simulink model "ALL_JP360_DBW_V6_5_1103"  (R2022a)
settings: Solver=FixedStepAuto  StartTime=0.0  StopTime=inf  FixedStep=0.01  RelTol=1e-3  EnableMultiTasking=on
model workspace (MAT data in the model file):
  g = 9.8
undefined symbols (not defined in the file or in its folder): canChannel, delta_v_p, IPM_Line_C0, IPM_Line_C1, IPM_Line_C2, IPM_Line_C3, M, M_p, MRR_ObjDistX, MRR_ObjDistY, MRR_ObjFusionCamID, MRR_ObjFusionSig, MRR_ObjID, MRR_ObjRelVelX, MRR_ObjRelVelY, MRR_ObjType, MRR_ObjUpdFlg, none, obj_vaild, untracktime, V, videoinput
libraries: canfdmsglib x230, canfdlib x76, slpidlib x24, simulink x18, dspstat3 x14, ctrlSharedLib x1, simulink_extras x1, imaqlib x1, realtime_pacer_lib x1, dspvision x1, visionsinks x1
(part 48 of 55)

== system ALL_JP360_DBW_V6_5_1103/MsgFromCAN/VR_ADCU_MsgFromCAN/VR_ADCU_MRR_Obj_25_26_0x69C ==
  VR_ADCU_MRR_Obj_25_26_0x69CFromInData : Inport  OutDataTypeStr=Bus:CAN_FD_MESSAGE_BUS
  Bus Creator : BusCreator  Inputs=30  OutDataTypeStr=Bus:VR_ADCU_MRR_Obj_25_26_0x69C  NonVirtualBus=on
  CAN FD Unpack : canfdmsglib/CAN FD Unpack  CANdbFile=HiFire_T360_P789_1R1V_Pri_Matrix_CAN_V2.3_20220810.dbc  MsgList=(none)  MsgName=MRR_Obj_25_26_0x69C  ProtocolMode=CAN FD  MsgIDType=Standard (11-bit identifier)  MsgIdentifier=1692  MsgLength=32  SignalInfo={'MRR_ObjDistX_25','26','12','BE','unsigned','Standard','0','0.0625','0','0','254.9375';'MRR_ObjDistX_26','130','12','BE','unsigned','Standard','0','0.0625','0','0','254.9375';'MRR_ObjDistY_25','44','14','BE','unsigned','Standard','0','0.0078125','-64','-64','63.9922';'MRR_ObjDistY_26','148','14','BE','unsigned','Standard','0','0.0078125','-64','-64','63.9922';'MRR_ObjExistProb_25','11','5','BE','unsigned','Standard','0','0.03125','0','0','0.96875';'MRR_ObjExistProb_26','115','5','BE','unsigned','Standard','0','0.03125','0','0','0.96875';'MRR_ObjFusionCamID_25','208','8','BE','unsigned','Standard','0','1','0','0','255';'MRR_ObjFusionCamID_26','216','8','BE','unsigned','Standard','0','1','0','0','255';'MRR_ObjFusionSig_25','98','2','BE','unsigned','Standard','0','1','0','0','3';'MRR_ObjFusionSig_26','202','2','BE','unsigned','Standard','0','1','0','0','3';'MRR_ObjID_25','0','8','BE','unsigned','Standard','0','1','0','0','255';'MRR_ObjID_26','104','8','BE','unsigned','Standard','0','1','0','0','255';'MRR_ObjMovingSts_25','103','3','BE','unsigned','Standard','0','1','0','0','7';'MRR_ObjMovingSts_26','207','3','BE','unsigned','Standard','0','1','0','0','7';'MRR_ObjObstacleProb_25','22','5','BE','unsigned','Standard','0','0.03125','0','0','0.96875';'MRR_ObjObstacleProb_26','126','5','BE','unsigned','Standard','0','0.03125','0','0','0.96875';'MRR_ObjRelAccelX_25','72','10','BE','unsigned','Standard','0','0.03125','-16','-16','15.9688';'MRR_ObjRelAccelX_26','176','10','BE','unsigned','Standard','0','0.03125','-16','-16','15.9688';'MRR_ObjRelAccelY_25','94','10','BE','unsigned','Standard','0','0.03125','-16','-16','15.9688';'MRR_ObjRelAccelY_26','198','10','BE','unsigned','Standard','0','0.03125','-16','-16','15.9688';'MRR_ObjRelVelX_25','63','13','BE','unsigned','Standard','0','0.03125','-128','-128','127.9688';'MRR_ObjRelVelX_26','167','13','BE','unsigned','Standard','0','0.03125','-128','-128','127.9688';'MRR_ObjRelVelY_25','66','13','BE','unsigned','Standard','0','0.03125','-128','-128','127.9688';'MRR_ObjRelVelY_26','170','13','BE','unsigned','Standard','0','0.03125','-128','-128','127.9688';'MRR_ObjType_25','90','4','BE','unsigned','Standard','0','1','0','0','15';'MRR_ObjType_26','194','4','BE','unsigned','Standard','0','1','0','0','15';'MRR_ObjUpdFlg_25','100','3','BE','unsigned','Standard','0','1','0','0','7';'MRR_ObjUpdFlg_26','204','3','BE','unsigned','Standard','0','1','0','0','7';'MRR_Obj_25_26_Checksum','248','16','BE','unsigned','Standard','0','1','0','0','65535';'MRR_Obj_25_26_MsgCounter','232','4','BE','unsigned','Standard','0','1','0','0','15'}  IDPort=off  TimestampPort=off  ErrorPort=off  RemotePort=off  LengthPort=off  StatusPort=off  BRSPort=off  ESIPort=off  DLCPort=off  ApplyMinMax=off
      settings: SourceProductBaseCode=ME,XP,VN  DataFormat=CANdb specified signals
  Data Type Conversion{1..6,15..24} (16 alike) : DataTypeConversion  OutDataTypeStr=single  SaturateOnIntegerOverflow=off  RndMeth=Floor
  Data Type Conversion{9..10,13..14,25..28,30} (9 alike) : DataTypeConversion  OutDataTypeStr=int8  SaturateOnIntegerOverflow=off  RndMeth=Floor
  Data Type Conversion{7..8,11..12} (4 alike) : DataTypeConversion  OutDataTypeStr=uint8  SaturateOnIntegerOverflow=off  RndMeth=Floor
  Data Type Conversion29 : DataTypeConversion  OutDataTypeStr=uint16  SaturateOnIntegerOverflow=off  RndMeth=Floor
  VR_ADCU_MRR_Obj_25_26_0x69CFromOutData : Outport  OutDataTypeStr=Bus:VR_ADCU_MRR_Obj_25_26_0x69C
  wires:
  CAN FD Unpack/1 -> Data Type Conversion1/1
  CAN FD Unpack/2 -> Data Type Conversion2/1
  CAN FD Unpack/3 -> Data Type Conversion3/1
  CAN FD Unpack/4 -> Data Type Conversion4/1
  CAN FD Unpack/5 -> Data Type Conversion5/1
  CAN FD Unpack/6 -> Data Type Conversion6/1
  CAN FD Unpack/7 -> Data Type Conversion7/1
  CAN FD Unpack/8 -> Data Type Conversion8/1
  CAN FD Unpack/9 -> Data Type Conversion9/1
  CAN FD Unpack/10 -> Data Type Conversion10/1
  CAN FD Unpack/11 -> Data Type Conversion11/1
  CAN FD Unpack/12 -> Data Type Conversion12/1
  CAN FD Unpack/13 -> Data Type Conversion13/1
  CAN FD Unpack/14 -> Data Type Conversion14/1
  CAN FD Unpack/15 -> Data Type Conversion15/1
  CAN FD Unpack/16 -> Data Type Conversion16/1
  CAN FD Unpack/17 -> Data Type Conversion17/1
  CAN FD Unpack/18 -> Data Type Conversion18/1
  CAN FD Unpack/19 -> Data Type Conversion19/1
  CAN FD Unpack/20 -> Data Type Conversion20/1
  CAN FD Unpack/21 -> Data Type Conversion21/1
  CAN FD Unpack/22 -> Data Type Conversion22/1
  CAN FD Unpack/23 -> Data Type Conversion23/1
  CAN FD Unpack/24 -> Data Type Conversion24/1
  CAN FD Unpack/25 -> Data Type Conversion25/1
  CAN FD Unpack/26 -> Data Type Conversion26/1
  CAN FD Unpack/27 -> Data Type Conversion27/1
  CAN FD Unpack/28 -> Data Type Conversion28/1
  CAN FD Unpack/29 -> Data Type Conversion29/1
  CAN FD Unpack/30 -> Data Type Conversion30/1
  Data Type Conversion1/1 -> Bus Creator/1  "MRR_ObjDistX_25"
  Data Type Conversion2/1 -> Bus Creator/2  "MRR_ObjDistX_26"
  Data Type Conversion3/1 -> Bus Creator/3  "MRR_ObjDistY_25"
  Data Type Conversion4/1 -> Bus Creator/4  "MRR_ObjDistY_26"
  Data Type Conversion5/1 -> Bus Creator/5  "MRR_ObjExistProb_25"
  Data Type Conversion6/1 -> Bus Creator/6  "MRR_ObjExistProb_26"
  Data Type Conversion7/1 -> Bus Creator/7  "MRR_ObjFusionCamID_25"
  Data Type Conversion8/1 -> Bus Creator/8  "MRR_ObjFusionCamID_26"
  Data Type Conversion9/1 -> Bus Creator/9  "MRR_ObjFusionSig_25"
  Data Type Conversion10/1 -> Bus Creator/10  "MRR_ObjFusionSig_26"
  Data Type Conversion11/1 -> Bus Creator/11  "MRR_ObjID_25"
  Data Type Conversion12/1 -> Bus Creator/12  "MRR_ObjID_26"
  Data Type Conversion13/1 -> Bus Creator/13  "MRR_ObjMovingSts_25"
  Data Type Conversion14/1 -> Bus Creator/14  "MRR_ObjMovingSts_26"
  Data Type Conversion15/1 -> Bus Creator/15  "MRR_ObjObstacleProb_25"
  Data Type Conversion16/1 -> Bus Creator/16  "MRR_ObjObstacleProb_26"
  Data Type Conversion17/1 -> Bus Creator/17  "MRR_ObjRelAccelX_25"
  Data Type Conversion18/1 -> Bus Creator/18  "MRR_ObjRelAccelX_26"
  Data Type Conversion19/1 -> Bus Creator/19  "MRR_ObjRelAccelY_25"
  Data Type Conversion20/1 -> Bus Creator/20  "MRR_ObjRelAccelY_26"
  Data Type Conversion21/1 -> Bus Creator/21  "MRR_ObjRelVelX_25"
  Data Type Conversion22/1 -> Bus Creator/22  "MRR_ObjRelVelX_26"
  Data Type Conversion23/1 -> Bus Creator/23  "MRR_ObjRelVelY_25"
  Data Type Conversion24/1 -> Bus Creator/24  "MRR_ObjRelVelY_26"
  Data Type Conversion25/1 -> Bus Creator/25  "MRR_ObjType_25"
  Data Type Conversion26/1 -> Bus Creator/26  "MRR_ObjType_26"
  Data Type Conversion27/1 -> Bus Creator/27  "MRR_ObjUpdFlg_25"
  Data Type Conversion28/1 -> Bus Creator/28  "MRR_ObjUpdFlg_26"
  Data Type Conversion29/1 -> Bus Creator/29  "MRR_Obj_25_26_Checksum"
  Data Type Conversion30/1 -> Bus Creator/30  "MRR_Obj_25_26_MsgCounter"
  Bus Creator/1 -> VR_ADCU_MRR_Obj_25_26_0x69CFromOutData/1  "VR_ADCU_MRR_Obj_25_26_0x69CFromOutData"
  VR_ADCU_MRR_Obj_25_26_0x69CFromInData/1 -> CAN FD Unpack/1  "VR_ADCU_MRR_Obj_25_26_0x69CFromInData"

== system ALL_JP360_DBW_V6_5_1103/MsgFromCAN/VR_ADCU_MsgFromCAN/VR_ADCU_MRR_Obj_27_28_0x69D ==
  VR_ADCU_MRR_Obj_27_28_0x69DFromInData : Inport  OutDataTypeStr=Bus:CAN_FD_MESSAGE_BUS
  Bus Creator : BusCreator  Inputs=30  OutDataTypeStr=Bus:VR_ADCU_MRR_Obj_27_28_0x69D  NonVirtualBus=on
  CAN FD Unpack : canfdmsglib/CAN FD Unpack  CANdbFile=HiFire_T360_P789_1R1V_Pri_Matrix_CAN_V2.3_20220810.dbc  MsgList=(none)  MsgName=MRR_Obj_27_28_0x69D  ProtocolMode=CAN FD  MsgIDType=Standard (11-bit identifier)  MsgIdentifier=1693  MsgLength=32  SignalInfo={'MRR_ObjDistX_27','26','12','BE','unsigned','Standard','0','0.0625','0','0','254.9375';'MRR_ObjDistX_28','130','12','BE','unsigned','Standard','0','0.0625','0','0','254.9375';'MRR_ObjDistY_27','44','14','BE','unsigned','Standard','0','0.0078125','-64','-64','63.9922';'MRR_ObjDistY_28','148','14','BE','unsigned','Standard','0','0.0078125','-64','-64','63.9922';'MRR_ObjExistProb_27','11','5','BE','unsigned','Standard','0','0.03125','0','0','0.96875';'MRR_ObjExistProb_28','115','5','BE','unsigned','Standard','0','0.03125','0','0','0.96875';'MRR_ObjFusionCamID_27','208','8','BE','unsigned','Standard','0','1','0','0','255';'MRR_ObjFusionCamID_28','216','8','BE','unsigned','Standard','0','1','0','0','255';'MRR_ObjFusionSig_27','98','2','BE','unsigned','Standard','0','1','0','0','3';'MRR_ObjFusionSig_28','202','2','BE','unsigned','Standard','0','1','0','0','3';'MRR_ObjID_27','0','8','BE','unsigned','Standard','0','1','0','0','255';'MRR_ObjID_28','104','8','BE','unsigned','Standard','0','1','0','0','255';'MRR_ObjMovingSts_27','103','3','BE','unsigned','Standard','0','1','0','0','7';'MRR_ObjMovingSts_28','207','3','BE','unsigned','Standard','0','1','0','0','7';'MRR_ObjObstacleProb_27','22','5','BE','unsigned','Standard','0','0.03125','0','0','0.96875';'MRR_ObjObstacleProb_28','126','5','BE','unsigned','Standard','0','0.03125','0','0','0.96875';'MRR_ObjRelAccelX_27','72','10','BE','unsigned','Standard','0','0.03125','-16','-16','15.9688';'MRR_ObjRelAccelX_28','176','10','BE','unsigned','Standard','0','0.03125','-16','-16','15.9688';'MRR_ObjRelAccelY_27','94','10','BE','unsigned','Standard','0','0.03125','-16','-16','15.9688';'MRR_ObjRelAccelY_28','198','10','BE','unsigned','Standard','0','0.03125','-16','-16','15.9688';'MRR_ObjRelVelX_27','63','13','BE','unsigned','Standard','0','0.03125','-128','-128','127.9688';'MRR_ObjRelVelX_28','167','13','BE','unsigned','Standard','0','0.03125','-128','-128','127.9688';'MRR_ObjRelVelY_27','66','13','BE','unsigned','Standard','0','0.03125','-128','-128','127.9688';'MRR_ObjRelVelY_28','170','13','BE','unsigned','Standard','0','0.03125','-128','-128','127.9688';'MRR_ObjType_27','90','4','BE','unsigned','Standard','0','1','0','0','15';'MRR_ObjType_28','194','4','BE','unsigned','Standard','0','1','0','0','15';'MRR_ObjUpdFlg_27','100','3','BE','unsigned','Standard','0','1','0','0','7';'MRR_ObjUpdFlg_28','204','3','BE','unsigned','Standard','0','1','0','0','7';'MRR_Obj_27_28_Checksum','248','16','BE','unsigned','Standard','0','1','0','0','65535';'MRR_Obj_27_28_MsgCounter','232','4','BE','unsigned','Standard','0','1','0','0','15'}  IDPort=off  TimestampPort=off  ErrorPort=off  RemotePort=off  LengthPort=off  StatusPort=off  BRSPort=off  ESIPort=off  DLCPort=off  ApplyMinMax=off
      settings: SourceProductBaseCode=ME,XP,VN  DataFormat=CANdb specified signals
  Data Type Conversion{1..6,15..24} (16 alike) : DataTypeConversion  OutDataTypeStr=single  SaturateOnIntegerOverflow=off  RndMeth=Floor
  Data Type Conversion{9..10,13..14,25..28,30} (9 alike) : DataTypeConversion  OutDataTypeStr=int8  SaturateOnIntegerOverflow=off  RndMeth=Floor
  Data Type Conversion{7..8,11..12} (4 alike) : DataTypeConversion  OutDataTypeStr=uint8  SaturateOnIntegerOverflow=off  RndMeth=Floor
  Data Type Conversion29 : DataTypeConversion  OutDataTypeStr=uint16  SaturateOnIntegerOverflow=off  RndMeth=Floor
  VR_ADCU_MRR_Obj_27_28_0x69DFromOutData : Outport  OutDataTypeStr=Bus:VR_ADCU_MRR_Obj_27_28_0x69D
  wires:
  CAN FD Unpack/1 -> Data Type Conversion1/1
  CAN FD Unpack/2 -> Data Type Conversion2/1
  CAN FD Unpack/3 -> Data Type Conversion3/1
  CAN FD Unpack/4 -> Data Type Conversion4/1
  CAN FD Unpack/5 -> Data Type Conversion5/1
  CAN FD Unpack/6 -> Data Type Conversion6/1
  CAN FD Unpack/7 -> Data Type Conversion7/1
  CAN FD Unpack/8 -> Data Type Conversion8/1
  CAN FD Unpack/9 -> Data Type Conversion9/1
  CAN FD Unpack/10 -> Data Type Conversion10/1
  CAN FD Unpack/11 -> Data Type Conversion11/1
  CAN FD Unpack/12 -> Data Type Conversion12/1
  CAN FD Unpack/13 -> Data Type Conversion13/1
  CAN FD Unpack/14 -> Data Type Conversion14/1
  CAN FD Unpack/15 -> Data Type Conversion15/1
  CAN FD Unpack/16 -> Data Type Conversion16/1
  CAN FD Unpack/17 -> Data Type Conversion17/1
  CAN FD Unpack/18 -> Data Type Conversion18/1
  CAN FD Unpack/19 -> Data Type Conversion19/1
  CAN FD Unpack/20 -> Data Type Conversion20/1
  CAN FD Unpack/21 -> Data Type Conversion21/1
  CAN FD Unpack/22 -> Data Type Conversion22/1
  CAN FD Unpack/23 -> Data Type Conversion23/1
  CAN FD Unpack/24 -> Data Type Conversion24/1
  CAN FD Unpack/25 -> Data Type Conversion25/1
  CAN FD Unpack/26 -> Data Type Conversion26/1
  CAN FD Unpack/27 -> Data Type Conversion27/1
  CAN FD Unpack/28 -> Data Type Conversion28/1
  CAN FD Unpack/29 -> Data Type Conversion29/1
  CAN FD Unpack/30 -> Data Type Conversion30/1
  Data Type Conversion1/1 -> Bus Creator/1  "MRR_ObjDistX_27"
  Data Type Conversion2/1 -> Bus Creator/2  "MRR_ObjDistX_28"
  Data Type Conversion3/1 -> Bus Creator/3  "MRR_ObjDistY_27"
  Data Type Conversion4/1 -> Bus Creator/4  "MRR_ObjDistY_28"
  Data Type Conversion5/1 -> Bus Creator/5  "MRR_ObjExistProb_27"
  Data Type Conversion6/1 -> Bus Creator/6  "MRR_ObjExistProb_28"
  Data Type Conversion7/1 -> Bus Creator/7  "MRR_ObjFusionCamID_27"
  Data Type Conversion8/1 -> Bus Creator/8  "MRR_ObjFusionCamID_28"
  Data Type Conversion9/1 -> Bus Creator/9  "MRR_ObjFusionSig_27"
  Data Type Conversion10/1 -> Bus Creator/10  "MRR_ObjFusionSig_28"
  Data Type Conversion11/1 -> Bus Creator/11  "MRR_ObjID_27"
  Data Type Conversion12/1 -> Bus Creator/12  "MRR_ObjID_28"
  Data Type Conversion13/1 -> Bus Creator/13  "MRR_ObjMovingSts_27"
  Data Type Conversion14/1 -> Bus Creator/14  "MRR_ObjMovingSts_28"
  Data Type Conversion15/1 -> Bus Creator/15  "MRR_ObjObstacleProb_27"
  Data Type Conversion16/1 -> Bus Creator/16  "MRR_ObjObstacleProb_28"
  Data Type Conversion17/1 -> Bus Creator/17  "MRR_ObjRelAccelX_27"
  Data Type Conversion18/1 -> Bus Creator/18  "MRR_ObjRelAccelX_28"
  Data Type Conversion19/1 -> Bus Creator/19  "MRR_ObjRelAccelY_27"
  Data Type Conversion20/1 -> Bus Creator/20  "MRR_ObjRelAccelY_28"
  Data Type Conversion21/1 -> Bus Creator/21  "MRR_ObjRelVelX_27"
  Data Type Conversion22/1 -> Bus Creator/22  "MRR_ObjRelVelX_28"
  Data Type Conversion23/1 -> Bus Creator/23  "MRR_ObjRelVelY_27"
  Data Type Conversion24/1 -> Bus Creator/24  "MRR_ObjRelVelY_28"
  Data Type Conversion25/1 -> Bus Creator/25  "MRR_ObjType_27"
  Data Type Conversion26/1 -> Bus Creator/26  "MRR_ObjType_28"
  Data Type Conversion27/1 -> Bus Creator/27  "MRR_ObjUpdFlg_27"
  Data Type Conversion28/1 -> Bus Creator/28  "MRR_ObjUpdFlg_28"
  Data Type Conversion29/1 -> Bus Creator/29  "MRR_Obj_27_28_Checksum"
  Data Type Conversion30/1 -> Bus Creator/30  "MRR_Obj_27_28_MsgCounter"
  Bus Creator/1 -> VR_ADCU_MRR_Obj_27_28_0x69DFromOutData/1  "VR_ADCU_MRR_Obj_27_28_0x69DFromOutData"
  VR_ADCU_MRR_Obj_27_28_0x69DFromInData/1 -> CAN FD Unpack/1  "VR_ADCU_MRR_Obj_27_28_0x69DFromInData"

== system ALL_JP360_DBW_V6_5_1103/MsgFromCAN/VR_ADCU_MsgFromCAN/VR_ADCU_MRR_Obj_29_30_0x69E ==
  VR_ADCU_MRR_Obj_29_30_0x69EFromInData : Inport  OutDataTypeStr=Bus:CAN_FD_MESSAGE_BUS
  Bus Creator : BusCreator  Inputs=30  OutDataTypeStr=Bus:VR_ADCU_MRR_Obj_29_30_0x69E  NonVirtualBus=on
  CAN FD Unpack : canfdmsglib/CAN FD Unpack  CANdbFile=HiFire_T360_P789_1R1V_Pri_Matrix_CAN_V2.3_20220810.dbc  MsgList=(none)  MsgName=MRR_Obj_29_30_0x69E  ProtocolMode=CAN FD  MsgIDType=Standard (11-bit identifier)  MsgIdentifier=1694  MsgLength=32  SignalInfo={'MRR_ObjDistX_29','26','12','BE','unsigned','Standard','0','0.0625','0','0','254.9375';'MRR_ObjDistX_30','130','12','BE','unsigned','Standard','0','0.0625','0','0','254.9375';'MRR_ObjDistY_29','44','14','BE','unsigned','Standard','0','0.0078125','-64','-64','63.9922';'MRR_ObjDistY_30','148','14','BE','unsigned','Standard','0','0.0078125','-64','-64','63.9922';'MRR_ObjExistProb_29','11','5','BE','unsigned','Standard','0','0.03125','0','0','0.96875';'MRR_ObjExistProb_30','115','5','BE','unsigned','Standard','0','0.03125','0','0','0.96875';'MRR_ObjFusionCamID_29','208','8','BE','unsigned','Standard','0','1','0','0','255';'MRR_ObjFusionCamID_30','216','8','BE','unsigned','Standard','0','1','0','0','255';'MRR_ObjFusionSig_29','98','2','BE','unsigned','Standard','0','1','0','0','3';'MRR_ObjFusionSig_30','202','2','BE','unsigned','Standard','0','1','0','0','3';'MRR_ObjID_29','0','8','BE','unsigned','Standard','0','1','0','0','255';'MRR_ObjID_30','104','8','BE','unsigned','Standard','0','1','0','0','255';'MRR_ObjMovingSts_29','103','3','BE','unsigned','Standard','0','1','0','0','7';'MRR_ObjMovingSts_30','207','3','BE','unsigned','Standard','0','1','0','0','7';'MRR_ObjObstacleProb_29','22','5','BE','unsigned','Standard','0','0.03125','0','0','0.96875';'MRR_ObjObstacleProb_30','126','5','BE','unsigned','Standard','0','0.03125','0','0','0.96875';'MRR_ObjRelAccelX_29','72','10','BE','unsigned','Standard','0','0.03125','-16','-16','15.9688';'MRR_ObjRelAccelX_30','176','10','BE','unsigned','Standard','0','0.03125','-16','-16','15.9688';'MRR_ObjRelAccelY_29','94','10','BE','unsigned','Standard','0','0.03125','-16','-16','15.9688';'MRR_ObjRelAccelY_30','198','10','BE','unsigned','Standard','0','0.03125','-16','-16','15.9688';'MRR_ObjRelVelX_29','63','13','BE','unsigned','Standard','0','0.03125','-128','-128','127.9688';'MRR_ObjRelVelX_30','167','13','BE','unsigned','Standard','0','0.03125','-128','-128','127.9688';'MRR_ObjRelVelY_29','66','13','BE','unsigned','Standard','0','0.03125','-128','-128','127.9688';'MRR_ObjRelVelY_30','170','13','BE','unsigned','Standard','0','0.03125','-128','-128','127.9688';'MRR_ObjType_29','90','4','BE','unsigned','Standard','0','1','0','0','15';'MRR_ObjType_30','194','4','BE','unsigned','Standard','0','1','0','0','15';'MRR_ObjUpdFlg_29','100','3','BE','unsigned','Standard','0','1','0','0','7';'MRR_ObjUpdFlg_30','204','3','BE','unsigned','Standard','0','1','0','0','7';'MRR_Obj_29_30_Checksum','248','16','BE','unsigned','Standard','0','1','0','0','65535';'MRR_Obj_29_30_MsgCounter','232','4','BE','unsigned','Standard','0','1','0','0','15'}  IDPort=off  TimestampPort=off  ErrorPort=off  RemotePort=off  LengthPort=off  StatusPort=off  BRSPort=off  ESIPort=off  DLCPort=off  ApplyMinMax=off
      settings: SourceProductBaseCode=ME,XP,VN  DataFormat=CANdb specified signals
  Data Type Conversion{1..6,15..24} (16 alike) : DataTypeConversion  OutDataTypeStr=single  SaturateOnIntegerOverflow=off  RndMeth=Floor
  Data Type Conversion{9..10,13..14,25..28,30} (9 alike) : DataTypeConversion  OutDataTypeStr=int8  SaturateOnIntegerOverflow=off  RndMeth=Floor
  Data Type Conversion{7..8,11..12} (4 alike) : DataTypeConversion  OutDataTypeStr=uint8  SaturateOnIntegerOverflow=off  RndMeth=Floor
  Data Type Conversion29 : DataTypeConversion  OutDataTypeStr=uint16  SaturateOnIntegerOverflow=off  RndMeth=Floor
  VR_ADCU_MRR_Obj_29_30_0x69EFromOutData : Outport  OutDataTypeStr=Bus:VR_ADCU_MRR_Obj_29_30_0x69E
  wires:
  CAN FD Unpack/1 -> Data Type Conversion1/1
  CAN FD Unpack/2 -> Data Type Conversion2/1
  CAN FD Unpack/3 -> Data Type Conversion3/1
  CAN FD Unpack/4 -> Data Type Conversion4/1
  CAN FD Unpack/5 -> Data Type Conversion5/1
  CAN FD Unpack/6 -> Data Type Conversion6/1
  CAN FD Unpack/7 -> Data Type Conversion7/1
  CAN FD Unpack/8 -> Data Type Conversion8/1
  CAN FD Unpack/9 -> Data Type Conversion9/1
  CAN FD Unpack/10 -> Data Type Conversion10/1
  CAN FD Unpack/11 -> Data Type Conversion11/1
  CAN FD Unpack/12 -> Data Type Conversion12/1
  CAN FD Unpack/13 -> Data Type Conversion13/1
  CAN FD Unpack/14 -> Data Type Conversion14/1
  CAN FD Unpack/15 -> Data Type Conversion15/1
  CAN FD Unpack/16 -> Data Type Conversion16/1
  CAN FD Unpack/17 -> Data Type Conversion17/1
  CAN FD Unpack/18 -> Data Type Conversion18/1
  CAN FD Unpack/19 -> Data Type Conversion19/1
  CAN FD Unpack/20 -> Data Type Conversion20/1
  CAN FD Unpack/21 -> Data Type Conversion21/1
  CAN FD Unpack/22 -> Data Type Conversion22/1
  CAN FD Unpack/23 -> Data Type Conversion23/1
  CAN FD Unpack/24 -> Data Type Conversion24/1
  CAN FD Unpack/25 -> Data Type Conversion25/1
  CAN FD Unpack/26 -> Data Type Conversion26/1
  CAN FD Unpack/27 -> Data Type Conversion27/1
  CAN FD Unpack/28 -> Data Type Conversion28/1
  CAN FD Unpack/29 -> Data Type Conversion29/1
  CAN FD Unpack/30 -> Data Type Conversion30/1
  Data Type Conversion1/1 -> Bus Creator/1  "MRR_ObjDistX_29"
  Data Type Conversion2/1 -> Bus Creator/2  "MRR_ObjDistX_30"
  Data Type Conversion3/1 -> Bus Creator/3  "MRR_ObjDistY_29"
  Data Type Conversion4/1 -> Bus Creator/4  "MRR_ObjDistY_30"
  Data Type Conversion5/1 -> Bus Creator/5  "MRR_ObjExistProb_29"
  Data Type Conversion6/1 -> Bus Creator/6  "MRR_ObjExistProb_30"
  Data Type Conversion7/1 -> Bus Creator/7  "MRR_ObjFusionCamID_29"
  Data Type Conversion8/1 -> Bus Creator/8  "MRR_ObjFusionCamID_30"
  Data Type Conversion9/1 -> Bus Creator/9  "MRR_ObjFusionSig_29"
  Data Type Conversion10/1 -> Bus Creator/10  "MRR_ObjFusionSig_30"
  Data Type Conversion11/1 -> Bus Creator/11  "MRR_ObjID_29"
  Data Type Conversion12/1 -> Bus Creator/12  "MRR_ObjID_30"
  Data Type Conversion13/1 -> Bus Creator/13  "MRR_ObjMovingSts_29"
  Data Type Conversion14/1 -> Bus Creator/14  "MRR_ObjMovingSts_30"
  Data Type Conversion15/1 -> Bus Creator/15  "MRR_ObjObstacleProb_29"
  Data Type Conversion16/1 -> Bus Creator/16  "MRR_ObjObstacleProb_30"
  Data Type Conversion17/1 -> Bus Creator/17  "MRR_ObjRelAccelX_29"
  Data Type Conversion18/1 -> Bus Creator/18  "MRR_ObjRelAccelX_30"
  Data Type Conversion19/1 -> Bus Creator/19  "MRR_ObjRelAccelY_29"
  Data Type Conversion20/1 -> Bus Creator/20  "MRR_ObjRelAccelY_30"
  Data Type Conversion21/1 -> Bus Creator/21  "MRR_ObjRelVelX_29"
  Data Type Conversion22/1 -> Bus Creator/22  "MRR_ObjRelVelX_30"
  Data Type Conversion23/1 -> Bus Creator/23  "MRR_ObjRelVelY_29"
  Data Type Conversion24/1 -> Bus Creator/24  "MRR_ObjRelVelY_30"
  Data Type Conversion25/1 -> Bus Creator/25  "MRR_ObjType_29"
  Data Type Conversion26/1 -> Bus Creator/26  "MRR_ObjType_30"
  Data Type Conversion27/1 -> Bus Creator/27  "MRR_ObjUpdFlg_29"
  Data Type Conversion28/1 -> Bus Creator/28  "MRR_ObjUpdFlg_30"
  Data Type Conversion29/1 -> Bus Creator/29  "MRR_Obj_29_30_Checksum"
  Data Type Conversion30/1 -> Bus Creator/30  "MRR_Obj_29_30_MsgCounter"
  Bus Creator/1 -> VR_ADCU_MRR_Obj_29_30_0x69EFromOutData/1  "VR_ADCU_MRR_Obj_29_30_0x69EFromOutData"
  VR_ADCU_MRR_Obj_29_30_0x69EFromInData/1 -> CAN FD Unpack/1  "VR_ADCU_MRR_Obj_29_30_0x69EFromInData"

== system ALL_JP360_DBW_V6_5_1103/MsgFromCAN/VR_ADCU_MsgFromCAN/VR_ADCU_MRR_Obj_31_32_0x69F ==
  VR_ADCU_MRR_Obj_31_32_0x69FFromInData : Inport  OutDataTypeStr=Bus:CAN_FD_MESSAGE_BUS
  Bus Creator : BusCreator  Inputs=30  OutDataTypeStr=Bus:VR_ADCU_MRR_Obj_31_32_0x69F  NonVirtualBus=on
  CAN FD Unpack : canfdmsglib/CAN FD Unpack  CANdbFile=HiFire_T360_P789_1R1V_Pri_Matrix_CAN_V2.3_20220810.dbc  MsgList=(none)  MsgName=MRR_Obj_31_32_0x69F  ProtocolMode=CAN FD  MsgIDType=Standard (11-bit identifier)  MsgIdentifier=1695  MsgLength=32  SignalInfo={'MRR_ObjDistX_31','26','12','BE','unsigned','Standard','0','0.0625','0','0','254.9375';'MRR_ObjDistX_32','130','12','BE','unsigned','Standard','0','0.0625','0','0','254.9375';'MRR_ObjDistY_31','44','14','BE','unsigned','Standard','0','0.0078125','-64','-64','63.9922';'MRR_ObjDistY_32','148','14','BE','unsigned','Standard','0','0.0078125','-64','-64','63.9922';'MRR_ObjExistProb_31','11','5','BE','unsigned','Standard','0','0.03125','0','0','0.96875';'MRR_ObjExistProb_32','115','5','BE','unsigned','Standard','0','0.03125','0','0','0.96875';'MRR_ObjFusionCamID_31','208','8','BE','unsigned','Standard','0','1','0','0','255';'MRR_ObjFusionCamID_32','216','8','BE','unsigned','Standard','0','1','0','0','255';'MRR_ObjFusionSig_31','98','2','BE','unsigned','Standard','0','1','0','0','3';'MRR_ObjFusionSig_32','202','2','BE','unsigned','Standard','0','1','0','0','3';'MRR_ObjID_31','0','8','BE','unsigned','Standard','0','1','0','0','255';'MRR_ObjID_32','104','8','BE','unsigned','Standard','0','1','0','0','255';'MRR_ObjMovingSts_31','103','3','BE','unsigned','Standard','0','1','0','0','7';'MRR_ObjMovingSts_32','207','3','BE','unsigned','Standard','0','1','0','0','7';'MRR_ObjObstacleProb_31','22','5','BE','unsigned','Standard','0','0.03125','0','0','0.96875';'MRR_ObjObstacleProb_32','126','5','BE','unsigned','Standard','0','0.03125','0','0','0.96875';'MRR_ObjRelAccelX_31','72','10','BE','unsigned','Standard','0','0.03125','-16','-16','15.9688';'MRR_ObjRelAccelX_32','176','10','BE','unsigned','Standard','0','0.03125','-16','-16','15.9688';'MRR_ObjRelAccelY_31','94','10','BE','unsigned','Standard','0','0.03125','-16','-16','15.9688';'MRR_ObjRelAccelY_32','198','10','BE','unsigned','Standard','0','0.03125','-16','-16','15.9688';'MRR_ObjRelVelX_31','63','13','BE','unsigned','Standard','0','0.03125','-128','-128','127.9688';'MRR_ObjRelVelX_32','167','13','BE','unsigned','Standard','0','0.03125','-128','-128','127.9688';'MRR_ObjRelVelY_31','66','13','BE','unsigned','Standard','0','0.03125','-128','-128','127.9688';'MRR_ObjRelVelY_32','170','13','BE','unsigned','Standard','0','0.03125','-128','-128','127.9688';'MRR_ObjType_31','90','4','BE','unsigned','Standard','0','1','0','0','15';'MRR_ObjType_32','194','4','BE','unsigned','Standard','0','1','0','0','15';'MRR_ObjUpdFlg_31','100','3','BE','unsigned','Standard','0','1','0','0','7';'MRR_ObjUpdFlg_32','204','3','BE','unsigned','Standard','0','1','0','0','7';'MRR_Obj_31_32_Checksum','248','16','BE','unsigned','Standard','0','1','0','0','65535';'MRR_Obj_31_32_MsgCounter','232','4','BE','unsigned','Standard','0','1','0','0','15'}  IDPort=off  TimestampPort=off  ErrorPort=off  RemotePort=off  LengthPort=off  StatusPort=off  BRSPort=off  ESIPort=off  DLCPort=off  ApplyMinMax=off
      settings: SourceProductBaseCode=ME,XP,VN  DataFormat=CANdb specified signals
  Data Type Conversion{1..6,15..24} (16 alike) : DataTypeConversion  OutDataTypeStr=single  SaturateOnIntegerOverflow=off  RndMeth=Floor
  Data Type Conversion{9..10,13..14,25..28,30} (9 alike) : DataTypeConversion  OutDataTypeStr=int8  SaturateOnIntegerOverflow=off  RndMeth=Floor
  Data Type Conversion{7..8,11..12} (4 alike) : DataTypeConversion  OutDataTypeStr=uint8  SaturateOnIntegerOverflow=off  RndMeth=Floor
  Data Type Conversion29 : DataTypeConversion  OutDataTypeStr=uint16  SaturateOnIntegerOverflow=off  RndMeth=Floor
  VR_ADCU_MRR_Obj_31_32_0x69FFromOutData : Outport  OutDataTypeStr=Bus:VR_ADCU_MRR_Obj_31_32_0x69F
  wires:
  CAN FD Unpack/1 -> Data Type Conversion1/1
  CAN FD Unpack/2 -> Data Type Conversion2/1
  CAN FD Unpack/3 -> Data Type Conversion3/1
  CAN FD Unpack/4 -> Data Type Conversion4/1
  CAN FD Unpack/5 -> Data Type Conversion5/1
  CAN FD Unpack/6 -> Data Type Conversion6/1
  CAN FD Unpack/7 -> Data Type Conversion7/1
  CAN FD Unpack/8 -> Data Type Conversion8/1
  CAN FD Unpack/9 -> Data Type Conversion9/1
  CAN FD Unpack/10 -> Data Type Conversion10/1
  CAN FD Unpack/11 -> Data Type Conversion11/1
  CAN FD Unpack/12 -> Data Type Conversion12/1
  CAN FD Unpack/13 -> Data Type Conversion13/1
  CAN FD Unpack/14 -> Data Type Conversion14/1
  CAN FD Unpack/15 -> Data Type Conversion15/1
  CAN FD Unpack/16 -> Data Type Conversion16/1
  CAN FD Unpack/17 -> Data Type Conversion17/1
  CAN FD Unpack/18 -> Data Type Conversion18/1
  CAN FD Unpack/19 -> Data Type Conversion19/1
  CAN FD Unpack/20 -> Data Type Conversion20/1
  CAN FD Unpack/21 -> Data Type Conversion21/1
  CAN FD Unpack/22 -> Data Type Conversion22/1
  CAN FD Unpack/23 -> Data Type Conversion23/1
  CAN FD Unpack/24 -> Data Type Conversion24/1
  CAN FD Unpack/25 -> Data Type Conversion25/1
  CAN FD Unpack/26 -> Data Type Conversion26/1
  CAN FD Unpack/27 -> Data Type Conversion27/1
  CAN FD Unpack/28 -> Data Type Conversion28/1
  CAN FD Unpack/29 -> Data Type Conversion29/1
  CAN FD Unpack/30 -> Data Type Conversion30/1
  Data Type Conversion1/1 -> Bus Creator/1  "MRR_ObjDistX_31"
  Data Type Conversion2/1 -> Bus Creator/2  "MRR_ObjDistX_32"
  Data Type Conversion3/1 -> Bus Creator/3  "MRR_ObjDistY_31"
  Data Type Conversion4/1 -> Bus Creator/4  "MRR_ObjDistY_32"
  Data Type Conversion5/1 -> Bus Creator/5  "MRR_ObjExistProb_31"
  Data Type Conversion6/1 -> Bus Creator/6  "MRR_ObjExistProb_32"
  Data Type Conversion7/1 -> Bus Creator/7  "MRR_ObjFusionCamID_31"
  Data Type Conversion8/1 -> Bus Creator/8  "MRR_ObjFusionCamID_32"
  Data Type Conversion9/1 -> Bus Creator/9  "MRR_ObjFusionSig_31"
  Data Type Conversion10/1 -> Bus Creator/10  "MRR_ObjFusionSig_32"
  Data Type Conversion11/1 -> Bus Creator/11  "MRR_ObjID_31"
  Data Type Conversion12/1 -> Bus Creator/12  "MRR_ObjID_32"
  Data Type Conversion13/1 -> Bus Creator/13  "MRR_ObjMovingSts_31"
  Data Type Conversion14/1 -> Bus Creator/14  "MRR_ObjMovingSts_32"
  Data Type Conversion15/1 -> Bus Creator/15  "MRR_ObjObstacleProb_31"
  Data Type Conversion16/1 -> Bus Creator/16  "MRR_ObjObstacleProb_32"
  Data Type Conversion17/1 -> Bus Creator/17  "MRR_ObjRelAccelX_31"
  Data Type Conversion18/1 -> Bus Creator/18  "MRR_ObjRelAccelX_32"
  Data Type Conversion19/1 -> Bus Creator/19  "MRR_ObjRelAccelY_31"
  Data Type Conversion20/1 -> Bus Creator/20  "MRR_ObjRelAccelY_32"
  Data Type Conversion21/1 -> Bus Creator/21  "MRR_ObjRelVelX_31"
  Data Type Conversion22/1 -> Bus Creator/22  "MRR_ObjRelVelX_32"
  Data Type Conversion23/1 -> Bus Creator/23  "MRR_ObjRelVelY_31"
  Data Type Conversion24/1 -> Bus Creator/24  "MRR_ObjRelVelY_32"
  Data Type Conversion25/1 -> Bus Creator/25  "MRR_ObjType_31"
  Data Type Conversion26/1 -> Bus Creator/26  "MRR_ObjType_32"
  Data Type Conversion27/1 -> Bus Creator/27  "MRR_ObjUpdFlg_31"
  Data Type Conversion28/1 -> Bus Creator/28  "MRR_ObjUpdFlg_32"
  Data Type Conversion29/1 -> Bus Creator/29  "MRR_Obj_31_32_Checksum"
  Data Type Conversion30/1 -> Bus Creator/30  "MRR_Obj_31_32_MsgCounter"
  Bus Creator/1 -> VR_ADCU_MRR_Obj_31_32_0x69FFromOutData/1  "VR_ADCU_MRR_Obj_31_32_0x69FFromOutData"
  VR_ADCU_MRR_Obj_31_32_0x69FFromInData/1 -> CAN FD Unpack/1  "VR_ADCU_MRR_Obj_31_32_0x69FFromInData"

== system ALL_JP360_DBW_V6_5_1103/MsgToCAN/CCAN_ADCU_MsgFromCAN/CCAN_ADCU_ADCU_0x538 ==
  Bus Creator : BusCreator  Inputs=2  OutDataTypeStr=Bus:CCAN_ADCU_ADCU_0x538  NonVirtualBus=on
  Data Type Conversion1 : DataTypeConversion  OutDataTypeStr=int8  SaturateOnIntegerOverflow=off  RndMeth=Floor
  Data Type Conversion2 : DataTypeConversion  OutDataTypeStr=boolean  SaturateOnIntegerOverflow=off  RndMeth=Floor
  CCAN_ADCU_ADCU_0x538FromOutData : Outport  OutDataTypeStr=Bus:CCAN_ADCU_ADCU_0x538
  wires:
  Data Type Conversion1/1 -> Bus Creator/1  "ADCU_state"
  Data Type Conversion2/1 -> Bus Creator/2  "BSD_FCTB_State"
  Bus Creator/1 -> CCAN_ADCU_ADCU_0x538FromOutData/1  "CCAN_ADCU_ADCU_0x538FromOutData"

== system ALL_JP360_DBW_V6_5_1103/MsgToCAN/CCAN_ADCU_MsgFromCAN/CCAN_ADCU_ADCU_CanTSyn_0x570 ==
  Bus Creator : BusCreator  Inputs=1  OutDataTypeStr=Bus:CCAN_ADCU_ADCU_CanTSyn_0x570  NonVirtualBus=on
  Data Type Conversion1 : DataTypeConversion  OutDataTypeStr=uint64  SaturateOnIntegerOverflow=off  RndMeth=Floor
  CCAN_ADCU_ADCU_CanTSyn_0x570FromOutData : Outport  OutDataTypeStr=Bus:CCAN_ADCU_ADCU_CanTSyn_0x570
  wires:
  Data Type Conversion1/1 -> Bus Creator/1  "CanTSyn"
  Bus Creator/1 -> CCAN_ADCU_ADCU_CanTSyn_0x570FromOutData/1  "CCAN_ADCU_ADCU_CanTSyn_0x570FromOutData"

== system ALL_JP360_DBW_V6_5_1103/MsgToCAN/CCAN_ADCU_MsgFromCAN/CCAN_ADCU_ADCU_DiagResp ==
  Bus Creator : BusCreator  Inputs=1  OutDataTypeStr=Bus:CCAN_ADCU_ADCU_DiagResp  NonVirtualBus=on
  Data Type Conversion1 : DataTypeConversion  OutDataTypeStr=uint64  SaturateOnIntegerOverflow=off  RndMeth=Floor
  CCAN_ADCU_ADCU_DiagRespFromOutData : Outport  OutDataTypeStr=Bus:CCAN_ADCU_ADCU_DiagResp
  wires:
  Data Type Conversion1/1 -> Bus Creator/1  "DiagRespFromADCU"
  Bus Creator/1 -> CCAN_ADCU_ADCU_DiagRespFromOutData/1  "CCAN_ADCU_ADCU_DiagRespFromOutData"

== system ALL_JP360_DBW_V6_5_1103/MsgToCAN/CCAN_ADCU_MsgFromCAN/CCAN_ADCU_IPM_0x245 ==
  IPM_LaneAssit_Status : Inport
  IPM_LaneAssit_TorqueReq : Inport  Port=2
  IPM_LaneAssit_TorqueReqStatus : Inport  Port=3
  line01 : Inport  Port=4
  line02 : Inport  Port=5
  Add : Sum  Inputs=+-
  Bus Creator : BusCreator  Inputs=21  OutDataTypeStr=Bus:CCAN_ADCU_IPM_0x245  NonVirtualBus=on
  Constant1 : Constant  Value=0  OutDataTypeStr=boolean
  Constant2 : Constant  Value=3  OutDataTypeStr=int8
  Constant3 : Constant  Value=5  OutDataTypeStr=int8
  Constant5 : Constant  Value=4  OutDataTypeStr=int8
  Constant6 : Constant  OutDataTypeStr=boolean
  Constant7 : Constant  Value=0  OutDataTypeStr=boolean
  Data Type Conversion1 : DataTypeConversion  OutDataTypeStr=uint8  SaturateOnIntegerOverflow=off  RndMeth=Floor
  Data Type Conversion{3,7,10,14..16,20} (7 alike) : DataTypeConversion  OutDataTypeStr=boolean  SaturateOnIntegerOverflow=off  RndMeth=Floor
  Data Type Conversion{2,4..6,8..9,11,13,18..19,21} (11 alike) : DataTypeConversion  OutDataTypeStr=int8  SaturateOnIntegerOverflow=off  RndMeth=Floor
  Data Type Conversion12 : DataTypeConversion  OutDataTypeStr=single  SaturateOnIntegerOverflow=off  RndMeth=Floor
  Data Type Conversion17 : DataTypeConversion  OutDataTypeStr=uint8  SaturateOnIntegerOverflow=off  RndMeth=Floor
  Rolling_Counter : simulink/User-Defined Functions/Rolling_Counter  SystemSampleTime=-1  VariantActivationTime=update diagram  Latency=0  AutoFrameSizeCalculation=off
      settings: SourceProductBaseCode=SL
  Switch : Switch  Criteria=u2 > Threshold  SaturateOnIntegerOverflow=off  InputSameDT=off
  Switch3 : Switch  Criteria=u2 ~= 0  SaturateOnIntegerOverflow=off  InputSameDT=off
  CCAN_ADCU_IPM_0x245FromOutData : Outport  OutDataTypeStr=Bus:CCAN_ADCU_IPM_0x245
  wires:
  Data Type Conversion1/1 -> Bus Creator/1  "Checksum_0x245"
  Data Type Conversion2/1 -> Bus Creator/2  "IPM_ADAS_Alerts"
  Data Type Conversion3/1 -> Bus Creator/3  "IPM_IHC_HighbeamReq"
  Data Type Conversion4/1 -> Bus Creator/4  "IPM_IHC_Status"
  Data Type Conversion5/1 -> Bus Creator/5  "IPM_LDWWarningType"
  Data Type Conversion6/1 -> Bus Creator/6  "IPM_LaneAssitType"
  Data Type Conversion7/1 -> Bus Creator/7  "IPM_LaneAssit_HandsonReq"
  Data Type Conversion8/1 -> Bus Creator/8  "IPM_LaneAssit_LeftVisualization"
  Data Type Conversion9/1 -> Bus Creator/9  "IPM_LaneAssit_RightVisualization"
  Data Type Conversion10/1 -> Bus Creator/10  "IPM_LaneAssit_Sensitivity"
  Data Type Conversion11/1 -> Bus Creator/11  "IPM_LaneAssit_Status"
  Data Type Conversion12/1 -> Bus Creator/12  "IPM_LaneAssit_TorqueReq"
  Data Type Conversion13/1 -> Bus Creator/13  "IPM_LaneAssit_TorqueReqStatus"
  Data Type Conversion14/1 -> Bus Creator/14  "IPM_LaneAssit_TorqueValidity"
  Data Type Conversion15/1 -> Bus Creator/15  "IPM_LaneAssit_WarningAudio"
  Data Type Conversion16/1 -> Bus Creator/16  "IPM_LaneAssit_WarningVibration"
  Data Type Conversion17/1 -> Bus Creator/17  "IPM_SLA_Spdlimit"
  Data Type Conversion18/1 -> Bus Creator/18  "IPM_SLA_SpdlimitUnits"
  Data Type Conversion19/1 -> Bus Creator/19  "IPM_SLA_Status"
  Data Type Conversion20/1 -> Bus Creator/20  "IPM_TJAICA_Status"
  Data Type Conversion21/1 -> Bus Creator/21  "RollingCounter_0x245"
  Bus Creator/1 -> CCAN_ADCU_IPM_0x245FromOutData/1  "CCAN_ADCU_IPM_0x245FromOutData"
  IPM_LaneAssit_TorqueReq/1 -> Data Type Conversion12/1
  Constant1/1 -> Data Type Conversion14/1
  Rolling_Counter/1 -> Data Type Conversion21/1
  IPM_LaneAssit_TorqueReqStatus/1 -> Data Type Conversion13/1
  Constant2/1 -> Switch/3
  Constant3/1 -> Switch/1
  IPM_LaneAssit_Status/1 -> Data Type Conversion11/1, Switch/2, Add/1
  Switch/1 -> Data Type Conversion6/1
  Constant5/1 -> Add/2
  Add/1 -> Switch3/2
  Constant6/1 -> Switch3/3
  Constant7/1 -> Switch3/1
  Switch3/1 -> Data Type Conversion20/1
  line01/1 -> Data Type Conversion8/1
  line02/1 -> Data Type Conversion9/1

== system ALL_JP360_DBW_V6_5_1103/MsgToCAN/CCAN_ADCU_MsgFromCAN/CCAN_ADCU_IPM_0x247 ==
  Bus Creator : BusCreator  Inputs=7  OutDataTypeStr=Bus:CCAN_ADCU_IPM_0x247  NonVirtualBus=on
  Data Type Conversion1 : DataTypeConversion  OutDataTypeStr=uint8  SaturateOnIntegerOverflow=off  RndMeth=Floor
  Data Type Conversion{2..4,6..7} (5 alike) : DataTypeConversion  OutDataTypeStr=int8  SaturateOnIntegerOverflow=off  RndMeth=Floor
  Data Type Conversion5 : DataTypeConversion  OutDataTypeStr=uint8  SaturateOnIntegerOverflow=off  RndMeth=Floor
  CCAN_ADCU_IPM_0x247FromOutData : Outport  OutDataTypeStr=Bus:CCAN_ADCU_IPM_0x247
  wires:
  Data Type Conversion1/1 -> Bus Creator/1  "Checksum_0x247"
  Data Type Conversion2/1 -> Bus Creator/2  "IPM_DCLCSts"
  Data Type Conversion3/1 -> Bus Creator/3  "IPM_DCLC_manualfeedback"
  Data Type Conversion4/1 -> Bus Creator/4  "IPM_ELKSts"
  Data Type Conversion5/1 -> Bus Creator/5  "IPM_Traffic_Sign_Dis"
  Data Type Conversion6/1 -> Bus Creator/6  "IPM_TurnIndicatorReq"
  Data Type Conversion7/1 -> Bus Creator/7  "RollingCounter_0x247"
  Bus Creator/1 -> CCAN_ADCU_IPM_0x247FromOutData/1  "CCAN_ADCU_IPM_0x247FromOutData"

== system ALL_JP360_DBW_V6_5_1103/MsgToCAN/CCAN_ADCU_MsgFromCAN/CCAN_ADCU_IPM_LeftLine_0x278 ==
  278 : Inport
  Bus Selector : BusSelector  OutputSignals=IPM_Line01_ViewRangeStart,IPM_Line01_ViewRangeEnd,IPM_Line01_C0,IPM_Line01_C3,IPM_Line01_C2,IPM_Line01_C1
  Bus Creator : BusCreator  Inputs=6  OutDataTypeStr=Bus:CCAN_ADCU_IPM_LeftLine_0x278  NonVirtualBus=on
  Data Type Conversion{1..6} (6 alike) : DataTypeConversion  OutDataTypeStr=single  SaturateOnIntegerOverflow=off  RndMeth=Floor
  CCAN_ADCU_IPM_LeftLine_0x278FromOutData : Outport  OutDataTypeStr=Bus:CCAN_ADCU_IPM_LeftLine_0x278
  wires:
  Data Type Conversion1/1 -> Bus Creator/1  "IPM_LedtLine_dx_start"
  Data Type Conversion2/1 -> Bus Creator/2  "IPM_LeftLine_dx_lookhead"
  Data Type Conversion3/1 -> Bus Creator/3  "IPM_LeftLine_dy"
  Data Type Conversion4/1 -> Bus Creator/4  "IPM_LeftLine_hor_curvature_alteration"
  Data Type Conversion5/1 -> Bus Creator/5  "IPM_LeftLine_hor_curve"
  Data Type Conversion6/1 -> Bus Creator/6  "IPM_LeftLine_yawangle"
  Bus Creator/1 -> CCAN_ADCU_IPM_LeftLine_0x278FromOutData/1  "CCAN_ADCU_IPM_LeftLine_0x278FromOutData"
  278/1 -> Bus Selector/1
  Bus Selector/3 -> Data Type Conversion3/1  "<IPM_Line01_C0>"
  Bus Selector/4 -> Data Type Conversion4/1  "<IPM_Line01_C3>"
  Bus Selector/2 -> Data Type Conversion2/1  "<IPM_Line01_ViewRangeEnd>"
  Bus Selector/5 -> Data Type Conversion5/1  "<IPM_Line01_C2>"
  Bus Selector/1 -> Data Type Conversion1/1  "<IPM_Line01_ViewRangeStart>"
  Bus Selector/6 -> Data Type Conversion6/1  "<IPM_Line01_C1>"

== system ALL_JP360_DBW_V6_5_1103/MsgToCAN/CCAN_ADCU_MsgFromCAN/CCAN_ADCU_IPM_LeftLine_0x280 ==
  In2 : Inport
  In1 : Inport  Port=2
  280 : Inport  Port=3
  Bus Selector : BusSelector  OutputSignals=IPM_Line03_Existence_Probability,IPM_Line03_ColorClass,IPM_Line03_Type,IPM_Line03_C3,IPM_Line03_C0,IPM_Line03_C2,IPM_Line03_C1
  Bus Creator : BusCreator  Inputs=9  OutDataTypeStr=Bus:CCAN_ADCU_IPM_LeftLine_0x280  NonVirtualBus=on
  Constant : Constant  OutDataTypeStr=int8
  Data Type Conversion{1..3,8..9} (5 alike) : DataTypeConversion  OutDataTypeStr=int8  SaturateOnIntegerOverflow=off  RndMeth=Floor
  Data Type Conversion{4..7} (4 alike) : DataTypeConversion  OutDataTypeStr=single  SaturateOnIntegerOverflow=off  RndMeth=Floor
  Switch : Switch  Criteria=u2 > Threshold  Threshold=0.5  SaturateOnIntegerOverflow=off  InputSameDT=off
  CCAN_ADCU_IPM_LeftLine_0x280FromOutData : Outport  OutDataTypeStr=Bus:CCAN_ADCU_IPM_LeftLine_0x280
  wires:
  Data Type Conversion1/1 -> Bus Creator/1  "IPM_LaneAssit_LeftLeftVisualization"
  Data Type Conversion2/1 -> Bus Creator/2  "IPM_LeftLeftLine_Color"
  Data Type Conversion3/1 -> Bus Creator/3  "IPM_LeftLeftLine_Type"
  Data Type Conversion4/1 -> Bus Creator/4  "IPM_LeftLeftLine_curvature_alteration"
  Data Type Conversion5/1 -> Bus Creator/5  "IPM_LeftLeftLine_dy"
  Data Type Conversion6/1 -> Bus Creator/6  "IPM_LeftLeftLine_hor_curve"
  Data Type Conversion7/1 -> Bus Creator/7  "IPM_LeftLeftLine_yawangle"
  Data Type Conversion8/1 -> Bus Creator/8  "IPM_LeftLine_Color"
  Data Type Conversion9/1 -> Bus Creator/9  "IPM_LeftLine_Type"
  Bus Creator/1 -> CCAN_ADCU_IPM_LeftLine_0x280FromOutData/1  "CCAN_ADCU_IPM_LeftLine_0x280FromOutData"
  280/1 -> Bus Selector/1
  Bus Selector/6 -> Data Type Conversion6/1  "<IPM_Line03_C2>"
  Bus Selector/5 -> Data Type Conversion5/1  "<IPM_Line03_C0>"
  Bus Selector/7 -> Data Type Conversion7/1  "<IPM_Line03_C1>"
  Bus Selector/4 -> Data Type Conversion4/1  "<IPM_Line03_C3>"
  Bus Selector/3 -> Data Type Conversion3/1  "<IPM_Line03_Type>"
  Bus Selector/2 -> Data Type Conversion2/1  "<IPM_Line03_ColorClass>"
  In1/1 -> Data Type Conversion8/1
  In2/1 -> Data Type Conversion9/1
  Constant/1 -> Switch/1
  Switch/1 -> Data Type Conversion1/1
  Bus Selector/1 -> Switch/2  "<IPM_Line03_Existence_Probability>"

== system ALL_JP360_DBW_V6_5_1103/MsgToCAN/CCAN_ADCU_MsgFromCAN/CCAN_ADCU_IPM_RightLine_0x490 ==
  490 : Inport
  Bus Selector : BusSelector  OutputSignals=IPM_Line02_ViewRangeEnd,IPM_Line02_ViewRangeStart,IPM_Line02_C0,IPM_Line02_C3,IPM_Line02_C2,IPM_Line02_C1
  Bus Creator : BusCreator  Inputs=6  OutDataTypeStr=Bus:CCAN_ADCU_IPM_RightLine_0x490  NonVirtualBus=on
  Data Type Conversion{1..6} (6 alike) : DataTypeConversion  OutDataTypeStr=single  SaturateOnIntegerOverflow=off  RndMeth=Floor
  CCAN_ADCU_IPM_RightLine_0x490FromOutData : Outport  OutDataTypeStr=Bus:CCAN_ADCU_IPM_RightLine_0x490
  wires:
  Data Type Conversion1/1 -> Bus Creator/1  "IPM_RightLine_dx_lookhead"
  Data Type Conversion2/1 -> Bus Creator/2  "IPM_RightLine_dx_start"
  Data Type Conversion3/1 -> Bus Creator/3  "IPM_RightLine_dy"
  Data Type Conversion4/1 -> Bus Creator/4  "IPM_RightLine_hor_curvature_alteration"
  Data Type Conversion5/1 -> Bus Creator/5  "IPM_RightLine_hor_curve"
  Data Type Conversion6/1 -> Bus Creator/6  "IPM_RightLine_yawangle"
  Bus Creator/1 -> CCAN_ADCU_IPM_RightLine_0x490FromOutData/1  "CCAN_ADCU_IPM_RightLine_0x490FromOutData"
  490/1 -> Bus Selector/1
  Bus Selector/4 -> Data Type Conversion4/1  "<IPM_Line02_C3>"
  Bus Selector/3 -> Data Type Conversion3/1  "<IPM_Line02_C0>"
  Bus Selector/5 -> Data Type Conversion5/1  "<IPM_Line02_C2>"
  Bus Selector/2 -> Data Type Conversion2/1  "<IPM_Line02_ViewRangeStart>"
  Bus Selector/6 -> Data Type Conversion6/1  "<IPM_Line02_C1>"
  Bus Selector/1 -> Data Type Conversion1/1  "<IPM_Line02_ViewRangeEnd>"

== system ALL_JP360_DBW_V6_5_1103/MsgToCAN/CCAN_ADCU_MsgFromCAN/CCAN_ADCU_IPM_RightLine_0x491 ==
  In2 : Inport
  In1 : Inport  Port=2
  491 : Inport  Port=3
  Bus Selector : BusSelector  OutputSignals=IPM_Line04_Existence_Probability,IPM_Line04_ColorClass,IPM_Line04_Type,IPM_Line04_C3,IPM_Line04_C0,IPM_Line04_C2,IPM_Line04_C1
  Bus Creator : BusCreator  Inputs=9  OutDataTypeStr=Bus:CCAN_ADCU_IPM_RightLine_0x491  NonVirtualBus=on
  Constant : Constant  OutDataTypeStr=int8
  Data Type Conversion{1..5} (5 alike) : DataTypeConversion  OutDataTypeStr=int8  SaturateOnIntegerOverflow=off  RndMeth=Floor
  Data Type Conversion{6..9} (4 alike) : DataTypeConversion  OutDataTypeStr=single  SaturateOnIntegerOverflow=off  RndMeth=Floor
  Switch : Switch  Criteria=u2 > Threshold  Threshold=0.5  SaturateOnIntegerOverflow=off  InputSameDT=off
  CCAN_ADCU_IPM_RightLine_0x491FromOutData : Outport  OutDataTypeStr=Bus:CCAN_ADCU_IPM_RightLine_0x491
  wires:
  Data Type Conversion1/1 -> Bus Creator/1  "IPM_LaneAssit_RightRightVisualization"
  Data Type Conversion2/1 -> Bus Creator/2  "IPM_RighRightLine_Color"
  Data Type Conversion3/1 -> Bus Creator/3  "IPM_RightLine_Color"
  Data Type Conversion4/1 -> Bus Creator/4  "IPM_RightLine_Type"
  Data Type Conversion5/1 -> Bus Creator/5  "IPM_RightRighLine_Type"
  Data Type Conversion6/1 -> Bus Creator/6  "IPM_RightRightLine_curvature_alteration"
  Data Type Conversion7/1 -> Bus Creator/7  "IPM_RightRightLine_dy"
  Data Type Conversion8/1 -> Bus Creator/8  "IPM_RightRightLine_hor_curve"
  Data Type Conversion9/1 -> Bus Creator/9  "IPM_RightRightLine_yawangle"
  Bus Creator/1 -> CCAN_ADCU_IPM_RightLine_0x491FromOutData/1  "CCAN_ADCU_IPM_RightLine_0x491FromOutData"
  491/1 -> Bus Selector/1
  In1/1 -> Data Type Conversion4/1
  In2/1 -> Data Type Conversion3/1
  Bus Selector/1 -> Switch/2  "<IPM_Line04_Existence_Probability>"
  Constant/1 -> Switch/1
  Switch/1 -> Data Type Conversion1/1
  Bus Selector/2 -> Data Type Conversion2/1  "<IPM_Line04_ColorClass>"
  Bus Selector/7 -> Data Type Conversion9/1  "<IPM_Line04_C1>"
  Bus Selector/6 -> Data Type Conversion8/1  "<IPM_Line04_C2>"
  Bus Selector/5 -> Data Type Conversion7/1  "<IPM_Line04_C0>"
  Bus Selector/4 -> Data Type Conversion6/1  "<IPM_Line04_C3>"
  Bus Selector/3 -> Data Type Conversion5/1  "<IPM_Line04_Type>"

== system ALL_JP360_DBW_V6_5_1103/MsgToCAN/CCAN_ADCU_MsgFromCAN/CCAN_ADCU_IPM_VLC_0x293 ==
  ACC_Torque_Request : Inport
  ACC_Torque_Request_Status : Inport  Port=2
  Bus Creator : BusCreator  Inputs=4  OutDataTypeStr=Bus:CCAN_ADCU_IPM_VLC_0x293  NonVirtualBus=on
  Data Type Conversion1 : DataTypeConversion  OutDataTypeStr=single  SaturateOnIntegerOverflow=off  RndMeth=Floor
  Data Type Conversion2 : DataTypeConversion  OutDataTypeStr=boolean  SaturateOnIntegerOverflow=off  RndMeth=Floor
  Data Type Conversion3 : DataTypeConversion  OutDataTypeStr=uint8  SaturateOnIntegerOverflow=off  RndMeth=Floor
  Data Type Conversion4 : DataTypeConversion  OutDataTypeStr=int8  SaturateOnIntegerOverflow=off  RndMeth=Floor
  Rolling_Counter : simulink/User-Defined Functions/Rolling_Counter  SystemSampleTime=-1  VariantActivationTime=update diagram  Latency=0  AutoFrameSizeCalculation=off
      settings: SourceProductBaseCode=SL
  CCAN_ADCU_IPM_VLC_0x293FromOutData : Outport  OutDataTypeStr=Bus:CCAN_ADCU_IPM_VLC_0x293
  wires:
  Data Type Conversion1/1 -> Bus Creator/1  "ACC_Torque_Request"
  Data Type Conversion2/1 -> Bus Creator/2  "ACC_Torque_Request_Status"
  Data Type Conversion3/1 -> Bus Creator/3  "Checksum_0x293"
  Data Type Conversion4/1 -> Bus Creator/4  "RollingCounter_0x293"
  Bus Creator/1 -> CCAN_ADCU_IPM_VLC_0x293FromOutData/1  "CCAN_ADCU_IPM_VLC_0x293FromOutData"
  ACC_Torque_Request/1 -> Data Type Conversion1/1
  ACC_Torque_Request_Status/1 -> Data Type Conversion2/1
  Rolling_Counter/1 -> Data Type Conversion4/1

== system ALL_JP360_DBW_V6_5_1103/MsgToCAN/CCAN_ADCU_MsgFromCAN/CCAN_ADCU_MRR_0x238 ==
  ACC_TgtAx : Inport
  Bus Creator : BusCreator  Inputs=7  OutDataTypeStr=Bus:CCAN_ADCU_MRR_0x238  NonVirtualBus=on
  Data Type Conversion{1..5} (5 alike) : DataTypeConversion  OutDataTypeStr=single  SaturateOnIntegerOverflow=off  RndMeth=Floor
  Data Type Conversion6 : DataTypeConversion  OutDataTypeStr=uint8  SaturateOnIntegerOverflow=off  RndMeth=Floor
  Data Type Conversion7 : DataTypeConversion  OutDataTypeStr=int8  SaturateOnIntegerOverflow=off  RndMeth=Floor
  Rolling_Counter : simulink/User-Defined Functions/Rolling_Counter  SystemSampleTime=-1  VariantActivationTime=update diagram  Latency=0  AutoFrameSizeCalculation=off
      settings: SourceProductBaseCode=SL
  CCAN_ADCU_MRR_0x238FromOutData : Outport  OutDataTypeStr=Bus:CCAN_ADCU_MRR_0x238
  wires:
  Data Type Conversion1/1 -> Bus Creator/1  "ACC_TgtAx"
  Data Type Conversion2/1 -> Bus Creator/2  "ACC_TgtAxLowerComftBand"
  Data Type Conversion3/1 -> Bus Creator/3  "ACC_TgtAxLowerLim"
  Data Type Conversion4/1 -> Bus Creator/4  "ACC_TgtAxUpperComftBand"
  Data Type Conversion5/1 -> Bus Creator/5  "ACC_TgtAxUpperLim"
  Data Type Conversion6/1 -> Bus Creator/6  "Checksum_0x238"
  Data Type Conversion7/1 -> Bus Creator/7  "RollingCounter_0x238"
  Bus Creator/1 -> CCAN_ADCU_MRR_0x238FromOutData/1  "CCAN_ADCU_MRR_0x238FromOutData"
  Rolling_Counter/1 -> Data Type Conversion7/1
  ACC_TgtAx/1 -> Data Type Conversion1/1
